simulink model "sampleModel1945"  (R2023a)
settings: Solver=VariableStepAuto  StartTime=0.0  StopTime=10.0  RelTol=1e-3
libraries: hdlsllib x5, simulink x1
settings Model: Creator=user1  LastModifiedBy=user1

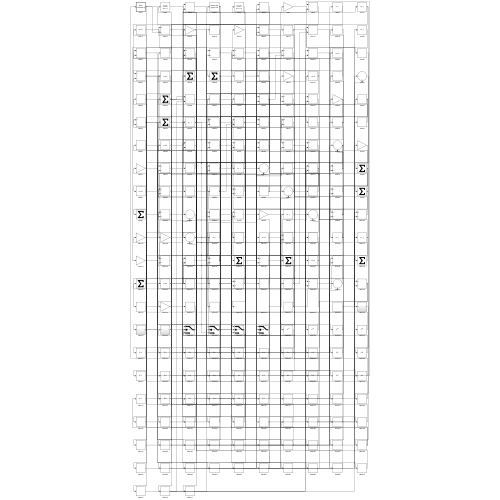
[thumbnail: Simulink's stored preview of the top-level diagram]
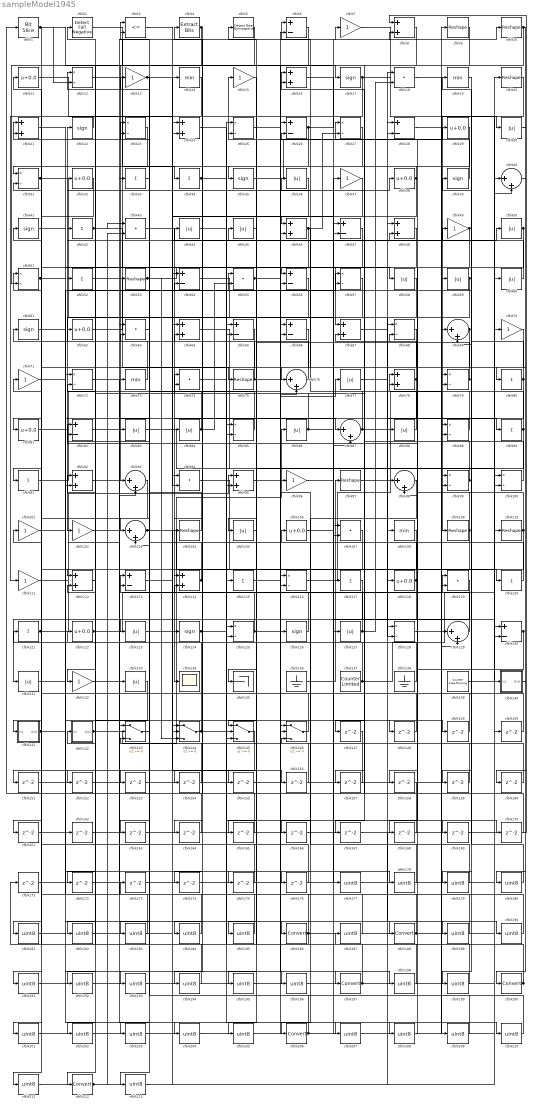
== system sampleModel1945 ==
  cfblk1 : hdlsllib/Logic and Bit Operations/Bit Slice  lidx=7  ridx=0
  cfblk{9..10,20,53,75,97,104,109..110} (9 alike) : Reshape
  cfblk{12,23,25,27,31,51,57,68,72,79,85,89,99..100,116,125,128} (17 alike) : Product  Inputs=*/  RndMeth=Zero  SaturateOnIntegerOverflow=on
  cfblk{7,13,15,37,49,70..71,96,101..102,111,132} (12 alike) : Gain
  cfblk{40,69,76,87,93,98,103,129} (8 alike) : Sum  Inputs=|++
  cfblk{30,36,44..45,50,58..60,77,83..84,86,88,105,123,127,131,133} (18 alike) : Abs  SaturateOnIntegerOverflow=off
  cfblk{11,29,32,38,62,81,106,118,122} (9 alike) : Bias  Bias=0.0  SaturateOnIntegerOverflow=off
  cfblk{18,43,55,63,74,94,107,119} (8 alike) : DotProduct  OutDataTypeStr=Inherit: Inherit via internal rule
  cfblk{14,19,73,108} (4 alike) : MinMax
  cfblk{8,16,21,24,46,48,64,67,78,92,95,112,114} (13 alike) : Sum
  cfblk{6,26,28,47,54,56,65..66,82,113,130} (11 alike) : Sum  Inputs=+-
  cfblk{33..34,42,52,80,90..91,115,117,120..121} (11 alike) : Sum  Inputs=+
  cfblk{17,22,35,39,41,61,124,126} (8 alike) : Signum
  cfblk134 : Scope
  cfblk135 : Terminator
  cfblk136 : Ground
  cfblk137 : hdlsllib/Sources/Counter Limited  uplimit=7  tsamp=-1
  cfblk138 : Ground
  cfblk139 : hdlsllib/Sources/Counter Free-Running  NumBits=16  tsamp=-1
  cfblk140 : Subsystem
      settings: LibrarySourceBlock=|
      | hdlsllib/Ports &
      | Subsystems/Subsystem
  cfblk141 : Subsystem
      settings: LibrarySourceBlock=|
      | hdlsllib/Ports &
      | Subsystems/Subsystem
  cfblk142 : Subsystem
      settings: LibrarySourceBlock=|
      | hdlsllib/Ports &
      | Subsystems/Subsystem
  cfblk{143..146} (4 alike) : Switch  SaturateOnIntegerOverflow=off  InputSameDT=off
  cfblk{147..176} (30 alike) : Delay  SampleTime=1
  cfblk{177..185,187,189..196,198..199,201..205,207..211,213} (31 alike) : DataTypeConversion  OutDataTypeStr=uint8  SaturateOnIntegerOverflow=off  RndMeth=Floor
  cfblk{186,188,197,200,206,212} (6 alike) : DataTypeConversion  SaturateOnIntegerOverflow=off  RndMeth=Floor
  cfblk2 : hdlsllib/Logic and Bit Operations/Detect Fall Negative  vinit=0  OutDataTypeStr=boolean
  cfblk3 : RelationalOperator  Operator=<=  OutDataTypeStr=boolean  InputSameDT=off
  cfblk4 : simulink/Logic and Bit Operations/Extract Bits  bitsToExtract=Upper half  numBits=8  bitIdxRange=[0 7]  outScalingMode=Preserve fixed-point scaling
      settings: LibrarySourceBlock=|
      | hdlsllib/Logic and Bit
      | Operations/Extract Bits
  cfblk5 : hdlsllib/Logic and Bit Operations/Detect Rise Nonnegative  vinit=0  OutDataTypeStr=boolean
  wires:
  cfblk38/1 -> cfblk35/1, cfblk94/2
  cfblk111/1 -> cfblk95/1
  cfblk20/1 -> cfblk109/1
  cfblk124/1 -> cfblk50/1, cfblk178/1
  cfblk55/1 -> cfblk38/1, cfblk155/1
  cfblk142/1(Out1) -> cfblk86/1, cfblk112/2
  cfblk114/1 -> cfblk21/1, cfblk112/1
  cfblk56/1 -> cfblk102/1
  cfblk89/1 -> cfblk78/1
  cfblk43/1 -> cfblk134/1
  cfblk105/1 -> cfblk55/1
  cfblk62/1 -> cfblk10/1
  cfblk65/1 -> cfblk114/1
  cfblk71/1 -> cfblk186/1
  cfblk94/1 -> cfblk120/1
  cfblk53/1 -> cfblk56/1, cfblk144/3
  cfblk136/1 -> cfblk97/1
  cfblk79/1 -> cfblk45/1, cfblk6/1
  cfblk10/1 -> cfblk80/1, cfblk192/1
  cfblk15/1 -> cfblk105/1
  cfblk113/1 -> cfblk48/2
  cfblk64/1 -> cfblk99/1
  cfblk48/1 -> cfblk67/1
  cfblk52/1 -> cfblk75/1
  cfblk40/1 -> cfblk200/1
  cfblk146/1 -> cfblk74/1
  cfblk123/1 -> cfblk119/1
  cfblk76/1 -> cfblk61/1
  cfblk75/1 -> cfblk51/1, cfblk27/1, cfblk165/1
  cfblk116/1 -> cfblk9/1
  cfblk12/1 -> cfblk34/1
  cfblk126/1 -> cfblk4/1
  cfblk23/1 -> cfblk31/1
  cfblk25/1 -> cfblk197/1
  cfblk120/1 -> cfblk12/1
  cfblk80/1 -> cfblk135/1, cfblk52/1, cfblk199/1
  cfblk110/1 -> cfblk68/2, cfblk166/1
  cfblk86/1 -> cfblk2/1, cfblk130/2, cfblk84/1
  cfblk8/1 -> cfblk93/1
  cfblk100/1 -> cfblk74/2
  cfblk132/1 -> cfblk133/1
  cfblk26/1 -> cfblk8/2, cfblk152/1
  cfblk74/1 -> cfblk65/1
  cfblk73/1 -> cfblk22/1
  cfblk141/1(Out1) -> cfblk121/1, cfblk57/2, cfblk207/1
  cfblk21/1 -> cfblk58/1
  cfblk108/1 -> cfblk212/1
  cfblk54/1 -> cfblk117/1
  cfblk69/1 -> cfblk92/2, cfblk213/1
  cfblk13/1 -> cfblk47/2, cfblk163/1
  cfblk46/1 -> cfblk76/1, cfblk91/1, cfblk27/2, cfblk153/1
  cfblk112/1 -> cfblk62/1
  cfblk22/1 -> cfblk111/1
  cfblk6/1 -> cfblk132/1
  cfblk129/1 -> cfblk113/1
  cfblk18/1 -> cfblk30/1
  cfblk130/1 -> cfblk158/1, cfblk159/1
  cfblk11/1 -> cfblk64/1
  cfblk118/1 -> cfblk3/1, cfblk172/1
  cfblk93/1 -> cfblk141/1(In1)
  cfblk7/1 -> cfblk140/1(In1)
  cfblk139/1 -> cfblk100/1
  cfblk5/1 -> cfblk73/1
  cfblk121/1 -> cfblk41/1, cfblk53/1
  cfblk49/1 -> cfblk124/1, cfblk168/1
  cfblk77/1 -> cfblk90/1
  cfblk95/1 -> cfblk146/2
  cfblk97/1 -> cfblk128/1
  cfblk33/1 -> cfblk83/1
  cfblk78/1 -> cfblk125/2, cfblk57/1, cfblk147/1
  cfblk34/1 -> cfblk184/1, cfblk198/1
  cfblk3/1 -> cfblk46/1
  cfblk91/1 -> cfblk54/1
  cfblk47/1 -> cfblk56/2
  cfblk109/1 -> cfblk26/2, cfblk82/2, cfblk123/1
  cfblk24/1 -> cfblk115/1
  cfblk50/1 -> cfblk145/3, cfblk167/1
  cfblk31/1 -> cfblk76/2, cfblk85/2
  cfblk67/1 -> cfblk118/1
  cfblk87/1 -> cfblk32/1, cfblk88/1
  cfblk59/1 -> cfblk39/1, cfblk154/1
  cfblk90/1 -> cfblk145/1, cfblk42/1
  cfblk122/1 -> cfblk94/1, cfblk6/2
  cfblk58/1 -> cfblk128/2
  cfblk17/1 -> cfblk79/2, cfblk104/1
  cfblk138/1 -> cfblk44/1
  cfblk128/1 -> cfblk89/2
  cfblk35/1 -> cfblk29/1
  cfblk84/1 -> cfblk13/1, cfblk55/2
  cfblk81/1 -> cfblk46/2
  cfblk102/1 -> cfblk33/1
  cfblk68/1 -> cfblk103/1
  cfblk83/1 -> cfblk130/1
  cfblk2/1 -> cfblk126/1
  cfblk72/1 -> cfblk188/1
  cfblk104/1 -> cfblk82/1
  cfblk103/1 -> cfblk116/2, cfblk156/1
  cfblk137/1 -> cfblk100/2, cfblk11/1, cfblk92/1
  cfblk143/1 -> cfblk103/2
  cfblk4/1 -> cfblk51/2, cfblk194/1
  cfblk125/1 -> cfblk23/1, cfblk77/1
  cfblk88/1 -> cfblk36/1
  cfblk51/1 -> cfblk145/2, cfblk196/1
  cfblk44/1 -> cfblk87/1
  cfblk119/1 -> cfblk131/1
  cfblk42/1 -> cfblk43/1, cfblk116/1, cfblk7/1, cfblk202/1
  cfblk1/1 -> cfblk17/1, cfblk81/1, cfblk12/2
  cfblk60/1 -> cfblk16/1
  cfblk127/1 -> cfblk96/1, cfblk18/2
  cfblk39/1 -> cfblk15/1
  cfblk144/1 -> cfblk49/1, cfblk122/1, cfblk169/1
  cfblk45/1 -> cfblk5/1
  cfblk85/1 -> cfblk64/2
  cfblk98/1 -> cfblk206/1
  cfblk99/1 -> cfblk16/2, cfblk69/2
  cfblk147/1 -> cfblk146/3
  cfblk61/1 -> cfblk148/1
  cfblk148/1 -> cfblk21/2
  cfblk16/1 -> cfblk149/1
  cfblk149/1 -> cfblk125/1
  cfblk150/1 -> cfblk78/2
  cfblk107/1 -> cfblk151/1
  cfblk151/1 -> cfblk69/1
  cfblk152/1 -> cfblk95/2
  cfblk153/1 -> cfblk99/2
  cfblk154/1 -> cfblk113/2
  cfblk155/1 -> cfblk48/1
  cfblk156/1 -> cfblk143/2
  cfblk9/1 -> cfblk157/1
  cfblk157/1 -> cfblk3/2
  cfblk158/1 -> cfblk1/1
  cfblk159/1 -> cfblk85/1
  cfblk30/1 -> cfblk160/1
  cfblk160/1 -> cfblk114/2
  cfblk145/1 -> cfblk161/1
  cfblk161/1 -> cfblk26/1
  cfblk131/1 -> cfblk162/1
  cfblk162/1 -> cfblk65/2
  cfblk163/1 -> cfblk79/1
  cfblk27/1 -> cfblk164/1
  cfblk164/1 -> cfblk23/2
  cfblk165/1 -> cfblk54/2
  cfblk166/1 -> cfblk89/1
  cfblk168/1 -> cfblk144/1
  cfblk169/1 -> cfblk8/1
  cfblk96/1 -> cfblk170/1
  cfblk170/1 -> cfblk67/2
  cfblk171/1 -> cfblk129/2
  cfblk172/1 -> cfblk93/2
  cfblk173/1 -> cfblk146/1
  cfblk36/1 -> cfblk174/1
  cfblk41/1 -> cfblk175/1
  cfblk175/1 -> cfblk24/1
  cfblk92/1 -> cfblk176/1
  cfblk176/1 -> cfblk31/2
  cfblk106/1 -> cfblk177/1
  cfblk177/1 -> cfblk110/1
  cfblk178/1 -> cfblk106/1
  cfblk19/1 -> cfblk179/1
  cfblk179/1 -> cfblk68/1
  cfblk140/1(Out1) -> cfblk180/1
  cfblk180/1 -> cfblk19/1
  cfblk14/1 -> cfblk181/1
  cfblk133/1 -> cfblk182/1
  cfblk182/1 -> cfblk14/1
  cfblk63/1 -> cfblk183/1
  cfblk183/1 -> cfblk143/1
  cfblk184/1 -> cfblk63/1
  cfblk29/1 -> cfblk185/1
  cfblk185/1 -> cfblk63/2
  cfblk186/1 -> cfblk171/1, cfblk144/2, cfblk60/1
  cfblk187/1 -> cfblk71/1
  cfblk188/1 -> cfblk20/1, cfblk107/1
  cfblk115/1 -> cfblk189/1
  cfblk189/1 -> cfblk72/1
  cfblk167/1 -> cfblk190/1
  cfblk190/1 -> cfblk72/2
  cfblk70/1 -> cfblk191/1
  cfblk191/1 -> cfblk107/2
  cfblk192/1 -> cfblk70/1
  cfblk101/1 -> cfblk193/1
  cfblk193/1 -> cfblk119/2
  cfblk194/1 -> cfblk101/1
  cfblk37/1 -> cfblk195/1
  cfblk195/1 -> cfblk59/1
  cfblk196/1 -> cfblk37/1
  cfblk197/1 -> cfblk18/1, cfblk47/1
  cfblk198/1 -> cfblk25/1
  cfblk199/1 -> cfblk25/2
  cfblk200/1 -> cfblk187/1, cfblk142/1(In1)
  cfblk117/1 -> cfblk201/1
  cfblk201/1 -> cfblk40/1
  cfblk202/1 -> cfblk40/2
  cfblk66/1 -> cfblk203/1
  cfblk203/1 -> cfblk127/1
  cfblk181/1 -> cfblk204/1
  cfblk204/1 -> cfblk66/1
  cfblk57/1 -> cfblk205/1
  cfblk205/1 -> cfblk66/2
  cfblk206/1 -> cfblk87/2, cfblk143/3, cfblk129/1
  cfblk207/1 -> cfblk98/1
  cfblk174/1 -> cfblk208/1
  cfblk208/1 -> cfblk98/2
  cfblk28/1 -> cfblk209/1
  cfblk209/1 -> cfblk173/1
  cfblk82/1 -> cfblk210/1
  cfblk210/1 -> cfblk28/1
  cfblk32/1 -> cfblk211/1
  cfblk211/1 -> cfblk28/2
  cfblk212/1 -> cfblk150/1, cfblk24/2, cfblk43/2
  cfblk213/1 -> cfblk108/1

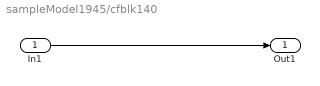
== system sampleModel1945/cfblk140 ==
  In1 : Inport
  Out1 : Outport
  wires:
  In1/1 -> Out1/1

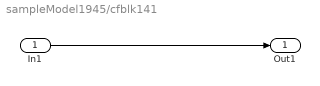
== system sampleModel1945/cfblk141 ==
  In1 : Inport
  Out1 : Outport
  wires:
  In1/1 -> Out1/1

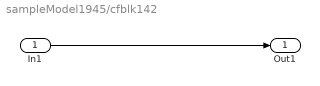
== system sampleModel1945/cfblk142 ==
  In1 : Inport
  Out1 : Outport
  wires:
  In1/1 -> Out1/1
